simulink model "DisplayModel"  (R2013b)
settings: Solver=FixedStepDiscrete  StartTime=0.0  StopTime=500  FixedStep=1  RelTol=1e-3
PostLoadFcn:
  | clear all;
  | close all;
  | delete(get(0,'Children'));
  | load busdata.mat;
  | load Input_data.mat;
StartFcn:
  | delete(get(0,'Children'));
  | sfcockpitDisplay;
undefined symbols (not defined in the file): AirplaneDirection, AirSpeed, Altitude, APUData, Bearing, CabinPressure, delete, Distance, ECAMInput, EFIS_Pressure, EPR, ExhaustTemp, FlapPosition, FlightAttitude, FuelPressure, FuelQuantity, GroundSpeed, h_ECAM, h_EFIS, h_FCU, h_ND, h_ND_AD, h_PFD_Pages, h_WEng, HydraulicPressure, LandingGear, NDPageInput, OilPressure, RateOfTurn, RPM, SelectedHeading, Temperature, VerticalSpeed
libraries: CockpitDisplayLib x35, aerolibanimutils x1, simulink x1
(part 1 of 2)
settings Model: CovPath=Control_and_Display_Logic/WarningManagement  CovHTMLOptions=-sRT=1 -aTS=1 -bRG=1 -bTC=1 -hTR=0 -nFC=0 -scm=1 -bcm=1 -xEv=0  Creator=siddhars  LastModifiedBy=siddhars
settings DataIOCC: SaveOutput=off  SaveTime=off
settings OptimizationCC: BlockReduction=off  ExpressionDepthLimit=2147483647  OptimizeModelRefInitCode=on  LifeSpan=1
settings DebuggingCC: ArrayBoundsChecking=error  MultiTaskDSMMsg=warning  MultiTaskCondExecSysMsg=none  BusObjectLabelMismatch=error  RootOutportRequireBusObject=error  StateNameClashWarn=warning  NonBusSignalsTreatedAsBus=error
settings RTWCC: SystemTargetFile=ert.tlc  GenCodeOnly=on  TemplateMakefile=ert_default_tmf  Description=Embedded Coder  GenerateReport=on  ProcessScript=ert_make_rtw_hook  IncludeHyperlinkInReport=on  LaunchReport=on  IncludeERTFirstTime=on  GenerateTraceInfo=on  GenerateTraceReport=on  GenerateTraceReportSl=on  GenerateTraceReportSf=on  GenerateTraceReportEml=on  GenerateWebview=on
settings CodeAppCC: IgnoreCustomStorageClasses=off  CustomSymbolStrType=$N$R$M  InternalIdentifier=Classic  ReqsInCode=on
settings ERTTargetCC: CodeReplacementLibrary=ANSI_C  GenerateSampleERTMain=on  SupportComplex=off  ERTCustomFileTemplate=example_file_process.tlc  EnableDataOwnership=on  MemSecPackage=Simulink
settings ConfigComp: Description=Design Verifier Custom Configuration Component  DVMode=DesignErrorDetection  DVMaxProcessTime=2000  DVModelCoverageObjectives=MCDC  DVMaxTestCaseSteps=1000  DVTestSuiteOptimization=CombinedObjectives (Nonlinear Extended)  DVCovFilter=on  DVDetectIntegerOverflow=off  DVDetectDivisionByZero=off  DVDetectDeadLogic=on  DVSaveReport=on  DVDisplayResultsOnModel=on

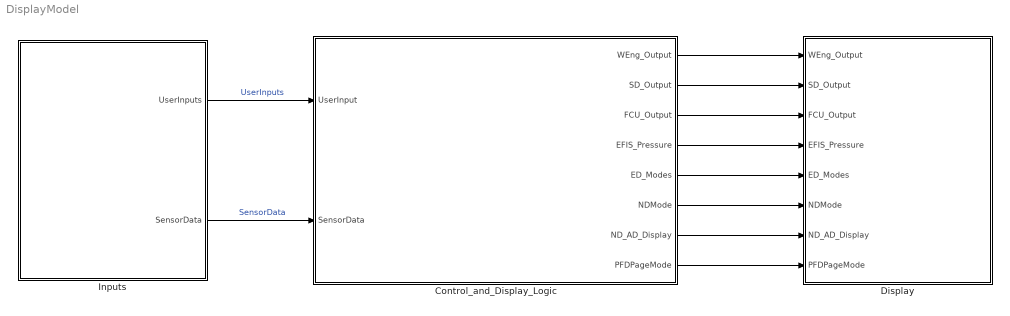
== system DisplayModel ==
  Control_and_Display_Logic : Subsystem  TreatAsAtomicUnit=on
  Display : Subsystem
  Inputs : Subsystem
  wires:
  Inputs/1(UserInputs) -> Control_and_Display_Logic/1(UserInput)  "UserInputs"
  Inputs/2(SensorData) -> Control_and_Display_Logic/2(SensorData)  "SensorData"
  Control_and_Display_Logic/2(SD_Output) -> Display/2(SD_Output)
  Control_and_Display_Logic/7(ND_AD_Display) -> Display/7(ND_AD_Display)
  Control_and_Display_Logic/3(FCU_Output) -> Display/3(FCU_Output)
  Control_and_Display_Logic/1(WEng_Output) -> Display/1(WEng_Output)
  Control_and_Display_Logic/6(NDMode) -> Display/6(NDMode)
  Control_and_Display_Logic/8(PFDPageMode) -> Display/8(PFDPageMode)
  Control_and_Display_Logic/5(ED_Modes) -> Display/5(ED_Modes)
  Control_and_Display_Logic/4(EFIS_Pressure) -> Display/4(EFIS_Pressure)

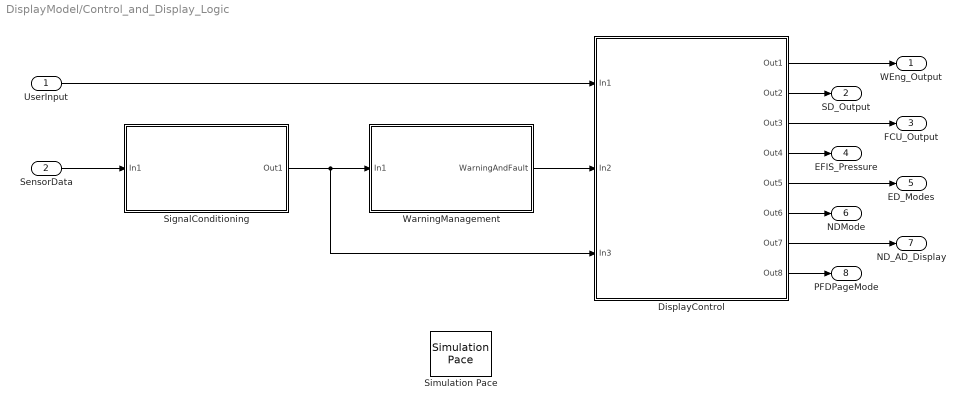
== system DisplayModel/Control_and_Display_Logic ==
  UserInput : Inport
  SensorData : Inport  Port=2
  DisplayControl : Subsystem
  SignalConditioning : Subsystem
  Simulation Pace : aerolibanimutils/Simulation Pace  SimulationPace=4  SleepMode=MATLAB Thread  OutputPaceError=off  SampleTime=1
      settings: AttributesFormatString=%<SimulationPace> sec/sec
  WarningManagement : Subsystem  TreatAsAtomicUnit=on
  WEng_Output : Outport
  SD_Output : Outport  Port=2
  FCU_Output : Outport  Port=3
  EFIS_Pressure : Outport  Port=4
  ED_Modes : Outport  Port=5
  NDMode : Outport  Port=6
  ND_AD_Display : Outport  Port=7
  PFDPageMode : Outport  Port=8
  wires:
  UserInput/1 -> DisplayControl/1(In1)
  SensorData/1 -> SignalConditioning/1(In1)
  SignalConditioning/1(Out1) -> WarningManagement/1(In1), DisplayControl/3(In3)
  DisplayControl/1(Out1) -> WEng_Output/1
  DisplayControl/2(Out2) -> SD_Output/1
  DisplayControl/3(Out3) -> FCU_Output/1
  DisplayControl/4(Out4) -> EFIS_Pressure/1
  DisplayControl/5(Out5) -> ED_Modes/1
  DisplayControl/6(Out6) -> NDMode/1
  DisplayControl/7(Out7) -> ND_AD_Display/1
  DisplayControl/8(Out8) -> PFDPageMode/1
  WarningManagement/1(WarningAndFault) -> DisplayControl/2(In2)

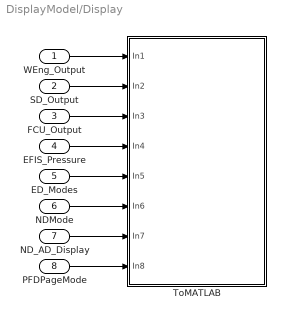
== system DisplayModel/Display ==
  WEng_Output : Inport
  SD_Output : Inport  Port=2
  FCU_Output : Inport  Port=3
  EFIS_Pressure : Inport  Port=4
  ED_Modes : Inport  Port=5
  NDMode : Inport  Port=6
  ND_AD_Display : Inport  Port=7
  PFDPageMode : Inport  Port=8
  ToMATLAB : Subsystem
  wires:
  PFDPageMode/1 -> ToMATLAB/8(In8)
  ND_AD_Display/1 -> ToMATLAB/7(In7)
  NDMode/1 -> ToMATLAB/6(In6)
  ED_Modes/1 -> ToMATLAB/5(In5)
  EFIS_Pressure/1 -> ToMATLAB/4(In4)
  FCU_Output/1 -> ToMATLAB/3(In3)
  SD_Output/1 -> ToMATLAB/2(In2)
  WEng_Output/1 -> ToMATLAB/1(In1)

== system DisplayModel/Inputs ==
  Sensors : Subsystem
  UserSelection : Subsystem
  UserInputs : Outport
  SensorData : Outport  Port=2
  wires:
  UserSelection/1(Out1) -> UserInputs/1
  UserSelection/2(Out2) -> Sensors/1(PowerSwitch)
  Sensors/1(SensorData) -> SensorData/1

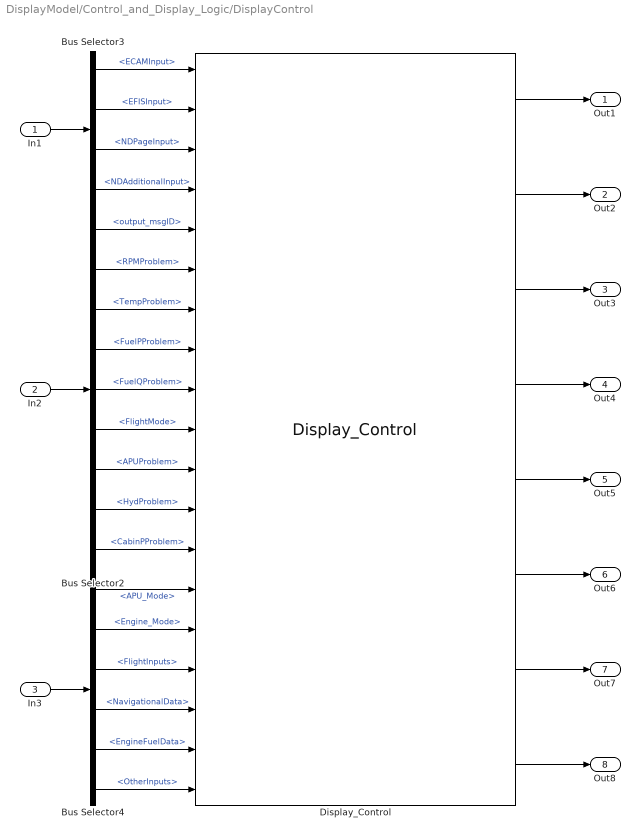
== system DisplayModel/Control_and_Display_Logic/DisplayControl ==
  In1 : Inport
  In2 : Inport  Port=2
  In3 : Inport  Port=3
  Bus Selector2 : BusSelector  OutputSignals=output_msgID,RPMProblem,TempProblem,FuelPProblem,FuelQProblem,FlightMode,APUProblem,HydProblem,CabinPProblem
  Bus Selector3 : BusSelector  OutputSignals=ECAMInput,EFISInput,NDPageInput,NDAdditionalInput
  Bus Selector4 : BusSelector  OutputSignals=EnergySystemModes.APU_Mode,EnergySystemModes.Engine_Mode,FlightInputs,NavigationalData,EngineFuelData,OtherInputs
  Display_Control : CockpitDisplayLib/Display_Control  SystemSampleTime=-1
  Out1 : Outport
  Out2 : Outport  Port=2
  Out3 : Outport  Port=3
  Out4 : Outport  Port=4
  Out5 : Outport  Port=5
  Out6 : Outport  Port=6
  Out7 : Outport  Port=7
  Out8 : Outport  Port=8
  wires:
  In2/1 -> Bus Selector2/1
  In3/1 -> Bus Selector4/1
  In1/1 -> Bus Selector3/1
  Bus Selector2/4 -> Display_Control/8  "<FuelPProblem>"
  Bus Selector2/3 -> Display_Control/7  "<TempProblem>"
  Display_Control/1 -> Out1/1
  Bus Selector2/8 -> Display_Control/12  "<HydProblem>"
  Bus Selector2/5 -> Display_Control/9  "<FuelQProblem>"
  Display_Control/8 -> Out8/1
  Display_Control/6 -> Out6/1
  Bus Selector2/6 -> Display_Control/10  "<FlightMode>"
  Bus Selector3/1 -> Display_Control/1  "<ECAMInput>"
  Display_Control/4 -> Out4/1
  Display_Control/3 -> Out3/1
  Bus Selector2/9 -> Display_Control/13  "<CabinPProblem>"
  Bus Selector3/2 -> Display_Control/2  "<EFISInput>"
  Display_Control/2 -> Out2/1
  Bus Selector2/2 -> Display_Control/6  "<RPMProblem>"
  Bus Selector3/3 -> Display_Control/3  "<NDPageInput>"
  Bus Selector3/4 -> Display_Control/4  "<NDAdditionalInput>"
  Bus Selector2/7 -> Display_Control/11  "<APUProblem>"
  Bus Selector2/1 -> Display_Control/5  "<output_msgID>"
  Display_Control/5 -> Out5/1
  Display_Control/7 -> Out7/1
  Bus Selector4/6 -> Display_Control/19  "<OtherInputs>"
  Bus Selector4/5 -> Display_Control/18  "<EngineFuelData>"
  Bus Selector4/4 -> Display_Control/17  "<NavigationalData>"
  Bus Selector4/3 -> Display_Control/16  "<FlightInputs>"
  Bus Selector4/2 -> Display_Control/15  "<Engine_Mode>"
  Bus Selector4/1 -> Display_Control/14  "<APU_Mode>"

== system DisplayModel/Control_and_Display_Logic/SignalConditioning ==
  In1 : Inport
  Bus Creator1 : BusCreator  Inputs=5
  Bus Selector6 : BusSelector  OutputSignals=EnergySystemModes,FlightInputs,NavigationalData,EngineFuelData,OtherInputs
  SignalSelection : Subsystem
  Out1 : Outport
  wires:
  Bus Selector6/2 -> Bus Creator1/2  "<FlightInputs>"
  Bus Creator1/1 -> Out1/1
  Bus Selector6/5 -> SignalSelection/2(In2)  "<OtherInputs>"
  Bus Selector6/4 -> SignalSelection/1(In1)  "<EngineFuelData>"
  Bus Selector6/3 -> Bus Creator1/3  "<NavigationalData>"
  SignalSelection/1(Out1) -> Bus Creator1/4  "EngineFuelData"
  In1/1 -> Bus Selector6/1
  SignalSelection/2(Out2) -> Bus Creator1/5  "OtherInputs"
  Bus Selector6/1 -> Bus Creator1/1  "<EnergySystemModes>"

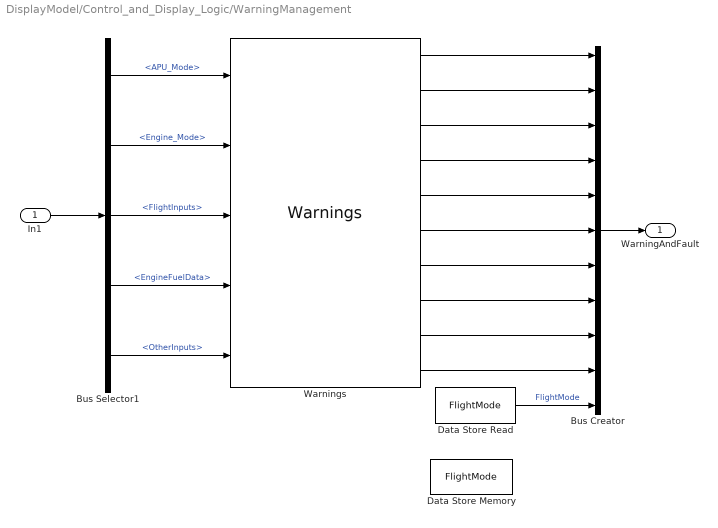
== system DisplayModel/Control_and_Display_Logic/WarningManagement ==
  In1 : Inport
  Bus Creator : BusCreator  Inputs=11
  Bus Selector1 : BusSelector  OutputSignals=EnergySystemModes.APU_Mode,EnergySystemModes.Engine_Mode,FlightInputs,EngineFuelData,OtherInputs
  Data Store Memory : DataStoreMemory  DataStoreName=FlightMode  ReadBeforeWriteMsg=warning  WriteAfterWriteMsg=warning  WriteAfterReadMsg=warning  OutDataTypeStr=double  Dimensions=1
  Data Store Read : DataStoreRead  Priority=1  DataStoreName=FlightMode  SampleTime=1
  Warnings : CockpitDisplayLib/Warnings  Priority=0  SystemSampleTime=-1
  WarningAndFault : Outport
  wires:
  In1/1 -> Bus Selector1/1
  Bus Creator/1 -> WarningAndFault/1
  Warnings/3 -> Bus Creator/3
  Warnings/6 -> Bus Creator/6
  Warnings/5 -> Bus Creator/5
  Warnings/4 -> Bus Creator/4
  Warnings/9 -> Bus Creator/9
  Warnings/7 -> Bus Creator/7
  Warnings/1 -> Bus Creator/1
  Warnings/10 -> Bus Creator/10
  Warnings/8 -> Bus Creator/8
  Warnings/2 -> Bus Creator/2
  Data Store Read/1 -> Bus Creator/11  "FlightMode"
  Bus Selector1/5 -> Warnings/5  "<OtherInputs>"
  Bus Selector1/4 -> Warnings/4  "<EngineFuelData>"
  Bus Selector1/3 -> Warnings/3  "<FlightInputs>"
  Bus Selector1/1 -> Warnings/1  "<APU_Mode>"
  Bus Selector1/2 -> Warnings/2  "<Engine_Mode>"

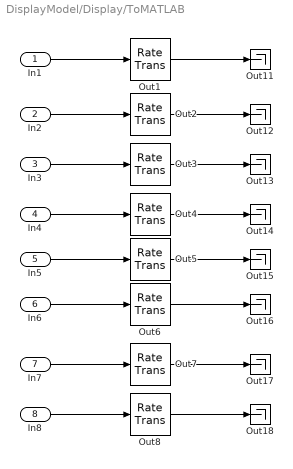
== system DisplayModel/Display/ToMATLAB ==
  In1 : Inport
  In2 : Inport  Port=2
  In3 : Inport  Port=3
  In4 : Inport  Port=4
  In5 : Inport  Port=5
  In6 : Inport  Port=6
  In7 : Inport  Port=7
  In8 : Inport  Port=8
  Out1 : RateTransition  StartFcn=|  StopFcn=delete(h_WEng)
      | blk='DisplayModel/Display/ToMATLAB/Out1';                                  
      | h_WEng=add_exec_event_listener(blk,'PostOutputs',@sfCockpitDisplay_helper);
  Out{11..18} (8 alike) : Terminator
  Out2 : RateTransition  StartFcn=|  StopFcn=delete(h_ECAM)
      | blk='DisplayModel/Display/ToMATLAB/Out2';                                  
      | h_ECAM=add_exec_event_listener(blk,'PostOutputs',@sfCockpitDisplay_helper);
  Out3 : RateTransition  StartFcn=|  StopFcn=delete(h_FCU)
      | blk='DisplayModel/Display/ToMATLAB/Out3';                                 
      | h_FCU=add_exec_event_listener(blk,'PostOutputs',@sfCockpitDisplay_helper);
  Out4 : RateTransition  StartFcn=|  StopFcn=delete(h_EFIS)
      | blk='DisplayModel/Display/ToMATLAB/Out4';                                  
      | h_EFIS=add_exec_event_listener(blk,'PostOutputs',@sfCockpitDisplay_helper);
  Out5 : RateTransition  StartFcn=|  StopFcn=|
      StartFcn=|
      | blk='DisplayModel/Display/ToMATLAB/Out5';                                  
      | h_ED_L=add_exec_event_listener(blk,'PostOutputs',@sfCockpitDisplay_helper);
      |                                                                            
      | h_ED_R=add_exec_event_listener(blk,'PostOutputs',@sfCockpitDisplay_helper);
      StopFcn=|
      | delete(h_ED_L)
      | delete(h_ED_R)
  Out6 : RateTransition  StartFcn=|  StopFcn=delete(h_ND)
      | blk='DisplayModel/Display/ToMATLAB/Out6';                                
      | h_ND=add_exec_event_listener(blk,'PostOutputs',@sfCockpitDisplay_helper);
  Out7 : RateTransition  StartFcn=|  StopFcn=delete(h_ND_AD)
      | blk='DisplayModel/Display/ToMATLAB/Out7';                                   
      | h_ND_AD=add_exec_event_listener(blk,'PostOutputs',@sfCockpitDisplay_helper);
  Out8 : RateTransition  StartFcn=|  StopFcn=delete(h_PFD_Pages)
      | blk='DisplayModel/Display/ToMATLAB/Out8';                                       
      | h_PFD_Pages=add_exec_event_listener(blk,'PostOutputs',@sfCockpitDisplay_helper);
  wires:
  Out1/1 -> Out11/1
  Out7/1 -> Out17/1
  Out5/1 -> Out15/1
  Out8/1 -> Out18/1
  Out6/1 -> Out16/1
  Out3/1 -> Out13/1
  Out2/1 -> Out12/1
  Out4/1 -> Out14/1
  In2/1 -> Out2/1
  In1/1 -> Out1/1
  In8/1 -> Out8/1
  In7/1 -> Out7/1
  In6/1 -> Out6/1
  In5/1 -> Out5/1
  In4/1 -> Out4/1
  In3/1 -> Out3/1

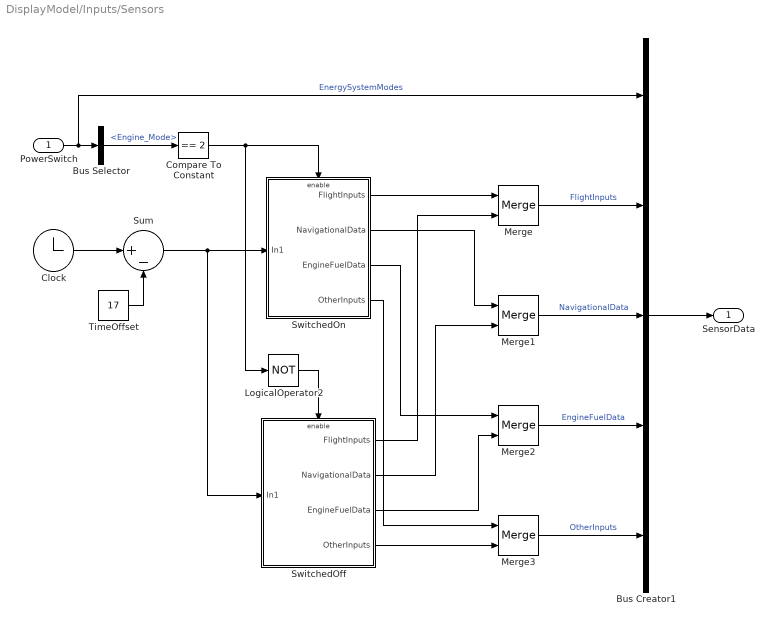
== system DisplayModel/Inputs/Sensors ==
  PowerSwitch : Inport
  Bus Creator1 : BusCreator  Inputs=5
  Bus Selector : BusSelector  OutputSignals=Engine_Mode
  Clock : Clock
  Compare To Constant : simulink/Logic and Bit Operations/Compare To Constant  relop===  const=2  OutDataTypeStr=boolean
  LogicalOperator2 : Logic  Operator=NOT  AllPortsSameDT=off  OutDataTypeStr=boolean
  Merge{,1..3} (4 alike) : Merge
  Sum : Sum  Inputs=|+-
  SwitchedOff : Subsystem
  SwitchedOn : Subsystem
  TimeOffset : Constant  Value=17
  SensorData : Outport
  wires:
  Clock/1 -> Sum/1
  Merge/1 -> Bus Creator1/2  "FlightInputs"
  SwitchedOff/1(FlightInputs) -> Merge/2
  SwitchedOn/4("OtherInputs ") -> Merge3/1
  SwitchedOff/3(EngineFuelData) -> Merge2/2
  SwitchedOff/2("NavigationalData ") -> Merge1/2
  SwitchedOn/1(FlightInputs) -> Merge/1
  SwitchedOn/2("NavigationalData ") -> Merge1/1
  Merge1/1 -> Bus Creator1/3  "NavigationalData"
  SwitchedOff/4("OtherInputs ") -> Merge3/2
  SwitchedOn/3(EngineFuelData) -> Merge2/1
  TimeOffset/1 -> Sum/2
  Sum/1 -> SwitchedOn/1(In1), SwitchedOff/1(In1)
  LogicalOperator2/1 -> SwitchedOff/Enable
  Bus Creator1/1 -> SensorData/1
  Merge2/1 -> Bus Creator1/4  "EngineFuelData"
  Merge3/1 -> Bus Creator1/5  "OtherInputs"
  PowerSwitch/1 -> Bus Selector/1, Bus Creator1/1  "EnergySystemModes"
  Bus Selector/1 -> Compare To Constant/1  "<Engine_Mode>"
  Compare To Constant/1 -> LogicalOperator2/1, SwitchedOn/Enable

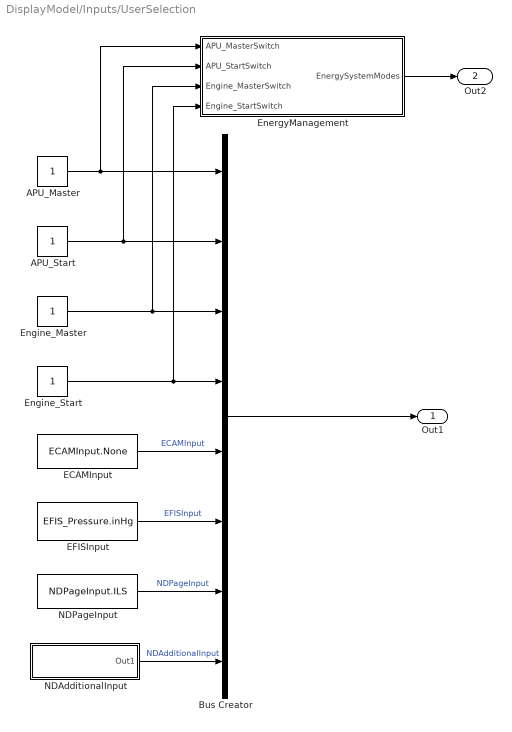
== system DisplayModel/Inputs/UserSelection ==
  APU_Master : Constant  OutDataTypeStr=boolean
  APU_Start : Constant  OutDataTypeStr=boolean
  Bus Creator : BusCreator  Inputs=8
  ECAMInput : Constant  Value=ECAMInput.None  OutDataTypeStr=Enum: ECAMInput
  EFISInput : Constant  Value=EFIS_Pressure.inHg  OutDataTypeStr=Enum: EFIS_Pressure
  EnergyManagement : Subsystem
  Engine_Master : Constant  OutDataTypeStr=boolean
  Engine_Start : Constant  OutDataTypeStr=boolean
  NDAdditionalInput : Subsystem
  NDPageInput : Constant  Value=NDPageInput.ILS  OutDataTypeStr=Enum: NDPageInput
  Out1 : Outport
  Out2 : Outport  Port=2
  wires:
  APU_Start/1 -> Bus Creator/2, EnergyManagement/2(APU_StartSwitch)
  Engine_Start/1 -> Bus Creator/4, EnergyManagement/4(Engine_StartSwitch)
  Engine_Master/1 -> Bus Creator/3, EnergyManagement/3(Engine_MasterSwitch)
  EFISInput/1 -> Bus Creator/6  "EFISInput"
  ECAMInput/1 -> Bus Creator/5  "ECAMInput"
  APU_Master/1 -> Bus Creator/1, EnergyManagement/1(APU_MasterSwitch)
  NDPageInput/1 -> Bus Creator/7  "NDPageInput"
  NDAdditionalInput/1(Out1) -> Bus Creator/8  "NDAdditionalInput"
  Bus Creator/1 -> Out1/1
  EnergyManagement/1(EnergySystemModes) -> Out2/1

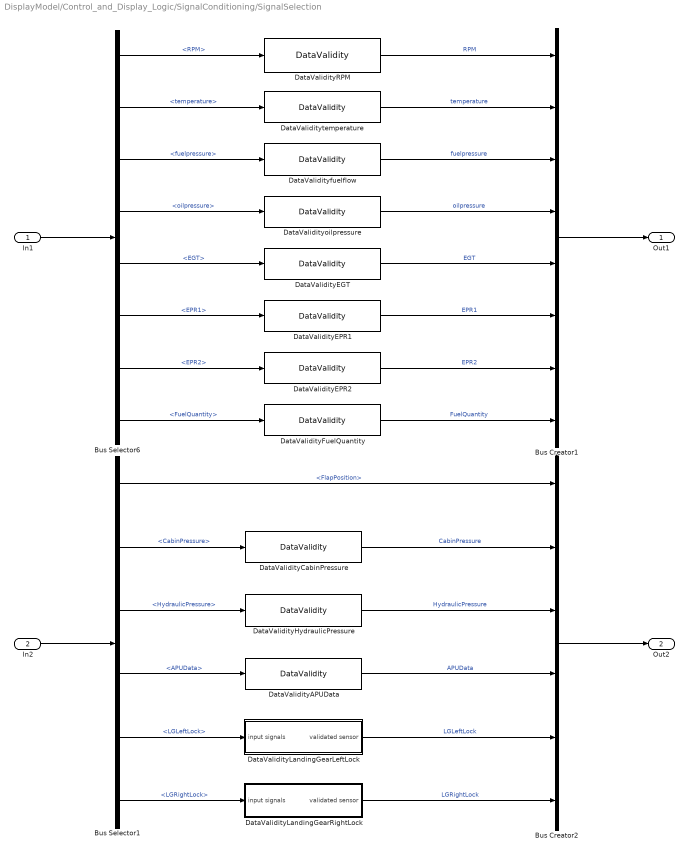
== system DisplayModel/Control_and_Display_Logic/SignalConditioning/SignalSelection ==
  In1 : Inport
  In2 : Inport  Port=2
  Bus Creator1 : BusCreator  Inputs=8  OutDataTypeStr=Bus: EngineFuel_Bus
  Bus Creator2 : BusCreator  Inputs=6  OutDataTypeStr=Bus: MiscData
  Bus Selector1 : BusSelector  OutputSignals=FlapPosition,CabinPressure,HydraulicPressure,APUData,LGLeftLock,LGRightLock
  Bus Selector6 : BusSelector  OutputSignals=RPM,temperature,fuelpressure,oilpressure,EGT,EPR1,EPR2,FuelQuantity
  DataValidityAPUData : CockpitDisplayLib/DataValidity
  DataValidityCabinPressure : CockpitDisplayLib/DataValidity
  DataValidityEGT : CockpitDisplayLib/DataValidity
  DataValidityEPR1 : CockpitDisplayLib/DataValidity
  DataValidityEPR2 : CockpitDisplayLib/DataValidity
  DataValidityFuelQuantity : CockpitDisplayLib/DataValidity
  DataValidityHydraulicPressure : CockpitDisplayLib/DataValidity
  DataValidityLandingGearLeftLock : Subsystem
  DataValidityLandingGearRightLock : Subsystem
  DataValidityRPM : CockpitDisplayLib/DataValidity
  DataValidityfuelflow : CockpitDisplayLib/DataValidity
  DataValidityoilpressure : CockpitDisplayLib/DataValidity
  DataValiditytemperature : CockpitDisplayLib/DataValidity
  Out1 : Outport
  Out2 : Outport  Port=2  OutDataTypeStr=Bus: MiscData
  wires:
  Bus Selector6/1 -> DataValidityRPM/1  "<RPM>"
  Bus Creator1/1 -> Out1/1
  DataValidityRPM/1 -> Bus Creator1/1  "RPM"
  Bus Selector6/6 -> DataValidityEPR1/1  "<EPR1>"
  In1/1 -> Bus Selector6/1
  Bus Selector6/4 -> DataValidityoilpressure/1  "<oilpressure>"
  Bus Selector6/5 -> DataValidityEGT/1  "<EGT>"
  Bus Selector6/3 -> DataValidityfuelflow/1  "<fuelpressure>"
  Bus Selector6/7 -> DataValidityEPR2/1  "<EPR2>"
  DataValidityoilpressure/1 -> Bus Creator1/4  "oilpressure"
  DataValidityfuelflow/1 -> Bus Creator1/3  "fuelpressure"
  DataValiditytemperature/1 -> Bus Creator1/2  "temperature"
  Bus Selector6/2 -> DataValiditytemperature/1  "<temperature>"
  In2/1 -> Bus Selector1/1
  Bus Creator2/1 -> Out2/1
  Bus Selector1/1 -> Bus Creator2/1  "<FlapPosition>"
  Bus Selector1/2 -> DataValidityCabinPressure/1  "<CabinPressure>"
  Bus Selector1/3 -> DataValidityHydraulicPressure/1  "<HydraulicPressure>"
  Bus Selector1/4 -> DataValidityAPUData/1  "<APUData>"
  Bus Selector1/5 -> DataValidityLandingGearLeftLock/1(input signals)  "<LGLeftLock>"
  DataValidityCabinPressure/1 -> Bus Creator2/2  "CabinPressure"
  DataValidityHydraulicPressure/1 -> Bus Creator2/3  "HydraulicPressure"
  DataValidityAPUData/1 -> Bus Creator2/4  "APUData"
  DataValidityLandingGearLeftLock/1(validated sensor) -> Bus Creator2/5  "LGLeftLock"
  DataValidityEGT/1 -> Bus Creator1/5  "EGT"
  DataValidityEPR1/1 -> Bus Creator1/6  "EPR1"
  DataValidityEPR2/1 -> Bus Creator1/7  "EPR2"
  Bus Selector6/8 -> DataValidityFuelQuantity/1  "<FuelQuantity>"
  DataValidityFuelQuantity/1 -> Bus Creator1/8  "FuelQuantity"
  DataValidityLandingGearRightLock/1(validated sensor) -> Bus Creator2/6  "LGRightLock"
  Bus Selector1/6 -> DataValidityLandingGearRightLock/1(input signals)  "<LGRightLock>"

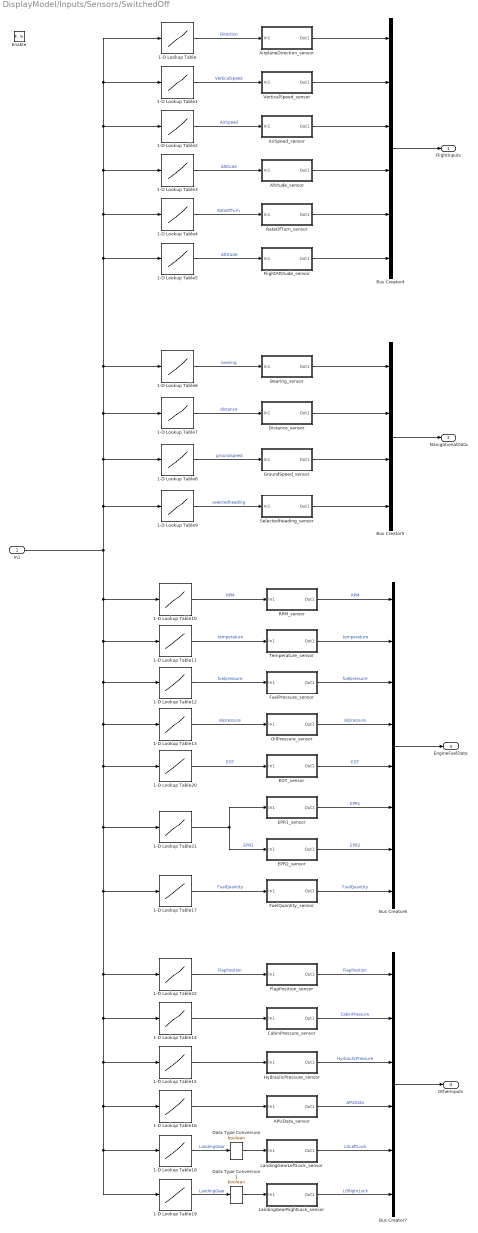
== system DisplayModel/Inputs/Sensors/SwitchedOff ==
  In1 : Inport
  Enable : EnablePort
  1-D Lookup Table{,1..17,20..22} (21 alike) : Lookup_n-D  NumberOfTableDimensions=1  BreakpointsForDimension1=0:10:500  Table=zeros(51,1)  RndMeth=Simplest  InputSameDT=on
  1-D Lookup Table18 : Lookup_n-D  NumberOfTableDimensions=1  BreakpointsForDimension1=0:10:500  Table=ones(51,1)  RndMeth=Simplest  InputSameDT=on
  1-D Lookup Table19 : Lookup_n-D  NumberOfTableDimensions=1  BreakpointsForDimension1=0:10:500  Table=ones(51,1)  RndMeth=Simplest  InputSameDT=on
  APUData_sensor : Subsystem
  AirSpeed_sensor : Subsystem
  AirplaneDirection_sensor : Subsystem
  Altitude_sensor : Subsystem
  Bearing_sensor : Subsystem
  Bus Creator4 : BusCreator  Inputs=6  OutDataTypeStr=Bus: FlightInputs
  Bus Creator5 : BusCreator  OutDataTypeStr=Bus: NavData
  Bus Creator6 : BusCreator  Inputs='RPM','temperature','fuelpressure','oilpressure','EGT','EPR1','EPR2','FuelQuantity'  OutDataTypeStr=Bus: IN_EngineFuel_Bus
  Bus Creator7 : BusCreator  Inputs=6  OutDataTypeStr=Bus: IN_MiscData
  CabinPressure_sensor : Subsystem
  Data Type Conversion : DataTypeConversion  OutDataTypeStr=boolean
  Data Type Conversion1 : DataTypeConversion  OutDataTypeStr=boolean
  Distance_sensor : Subsystem
  EGT_sensor : Subsystem
  EPR1_sensor : Subsystem
  EPR2_sensor : Subsystem
  FlapPosition_sensor : Subsystem
  FlightAttitude_sensor : Subsystem
  FuelPressure_sensor : Subsystem
  FuelQuantity_sensor : Subsystem
  GroundSpeed_sensor : Subsystem
  HydraulicPressure_sensor : Subsystem
  LandingGearLeftLock_sensor : Subsystem
  LandingGearRightLock_sensor : Subsystem
  OilPressure_sensor : Subsystem
  RPM_sensor : Subsystem
  RateOfTurn_sensor : Subsystem
  SelectedHeading_sensor : Subsystem
  Temperature_sensor : Subsystem
  VerticalSpeed_sensor : Subsystem
  FlightInputs : Outport
  "NavigationalData " : Outport  Port=2
  EngineFuelData : Outport  Port=3
  "OtherInputs " : Outport  Port=4
  wires:
  Bus Creator7/1 -> "OtherInputs "/1
  1-D Lookup Table22/1 -> FlapPosition_sensor/1(In1)  "FlapPosition"
  Bus Creator6/1 -> EngineFuelData/1
  1-D Lookup Table11/1 -> Temperature_sensor/1(In1)  "temperature"
  Bus Creator5/1 -> "NavigationalData "/1
  1-D Lookup Table9/1 -> SelectedHeading_sensor/1(In1)  "selectedheading"
  1-D Lookup Table8/1 -> GroundSpeed_sensor/1(In1)  "groundspeed"
  1-D Lookup Table6/1 -> Bearing_sensor/1(In1)  "bearing"
  1-D Lookup Table7/1 -> Distance_sensor/1(In1)  "distance"
  Bus Creator4/1 -> FlightInputs/1
  1-D Lookup Table5/1 -> FlightAttitude_sensor/1(In1)  "Attitude"
  1-D Lookup Table4/1 -> RateOfTurn_sensor/1(In1)  "RateOfTurn"
  1-D Lookup Table/1 -> AirplaneDirection_sensor/1(In1)  "Direction"
  1-D Lookup Table3/1 -> Altitude_sensor/1(In1)  "Altitude"
  1-D Lookup Table1/1 -> VerticalSpeed_sensor/1(In1)  "VerticalSpeed"
  1-D Lookup Table2/1 -> AirSpeed_sensor/1(In1)  "AirSpeed"
  1-D Lookup Table20/1 -> EGT_sensor/1(In1)  "EGT"
  1-D Lookup Table14/1 -> CabinPressure_sensor/1(In1)
  CabinPressure_sensor/1(Out1) -> Bus Creator7/2  "CabinPressure"
  1-D Lookup Table18/1 -> Data Type Conversion/1  "LandingGear"
  LandingGearLeftLock_sensor/1(Out1) -> Bus Creator7/5  "LGLeftLock"
  1-D Lookup Table16/1 -> APUData_sensor/1(In1)
  APUData_sensor/1(Out1) -> Bus Creator7/4  "APUData"
  1-D Lookup Table15/1 -> HydraulicPressure_sensor/1(In1)
  HydraulicPressure_sensor/1(Out1) -> Bus Creator7/3  "HydraulicPressure"
  EPR1_sensor/1(Out1) -> Bus Creator6/6  "EPR1"
  1-D Lookup Table13/1 -> OilPressure_sensor/1(In1)  "oilpressure"
  OilPressure_sensor/1(Out1) -> Bus Creator6/4  "oilpressure"
  1-D Lookup Table12/1 -> FuelPressure_sensor/1(In1)  "fuelpressure"
  FuelPressure_sensor/1(Out1) -> Bus Creator6/3  "fuelpressure"
  1-D Lookup Table10/1 -> RPM_sensor/1(In1)  "RPM"
  RPM_sensor/1(Out1) -> Bus Creator6/1  "RPM"
  Temperature_sensor/1(Out1) -> Bus Creator6/2  "temperature"
  SelectedHeading_sensor/1(Out1) -> Bus Creator5/4
  GroundSpeed_sensor/1(Out1) -> Bus Creator5/3
  Distance_sensor/1(Out1) -> Bus Creator5/2
  Bearing_sensor/1(Out1) -> Bus Creator5/1
  FlightAttitude_sensor/1(Out1) -> Bus Creator4/6
  RateOfTurn_sensor/1(Out1) -> Bus Creator4/5
  Altitude_sensor/1(Out1) -> Bus Creator4/4
  AirSpeed_sensor/1(Out1) -> Bus Creator4/3
  VerticalSpeed_sensor/1(Out1) -> Bus Creator4/2
  AirplaneDirection_sensor/1(Out1) -> Bus Creator4/1
  EGT_sensor/1(Out1) -> Bus Creator6/5  "EGT"
  FlapPosition_sensor/1(Out1) -> Bus Creator7/1  "FlapPosition"
  1-D Lookup Table21/1 -> EPR1_sensor/1(In1), EPR2_sensor/1(In1)  "EPR1"
  EPR2_sensor/1(Out1) -> Bus Creator6/7  "EPR2"
  1-D Lookup Table17/1 -> FuelQuantity_sensor/1(In1)  "FuelQuantity"
  FuelQuantity_sensor/1(Out1) -> Bus Creator6/8  "FuelQuantity"
  Data Type Conversion/1 -> LandingGearLeftLock_sensor/1(In1)
  1-D Lookup Table19/1 -> Data Type Conversion1/1  "LandingGear"
  LandingGearRightLock_sensor/1(Out1) -> Bus Creator7/6  "LGRightLock"
  In1/1 -> 1-D Lookup Table17/1, 1-D Lookup Table18/1, 1-D Lookup Table19/1, 1-D Lookup Table16/1, 1-D Lookup Table15/1, 1-D Lookup Table14/1, 1-D Lookup Table22/1, 1-D Lookup Table21/1, 1-D Lookup Table20/1, 1-D Lookup Table13/1, 1-D Lookup Table12/1, 1-D Lookup Table11/1, 1-D Lookup Table10/1, 1-D Lookup Table5/1, 1-D Lookup Table3/1, 1-D Lookup Table2/1, 1-D Lookup Table1/1, 1-D Lookup Table/1, 1-D Lookup Table4/1, 1-D Lookup Table6/1, 1-D Lookup Table7/1, 1-D Lookup Table8/1, 1-D Lookup Table9/1
  Data Type Conversion1/1 -> LandingGearRightLock_sensor/1(In1)

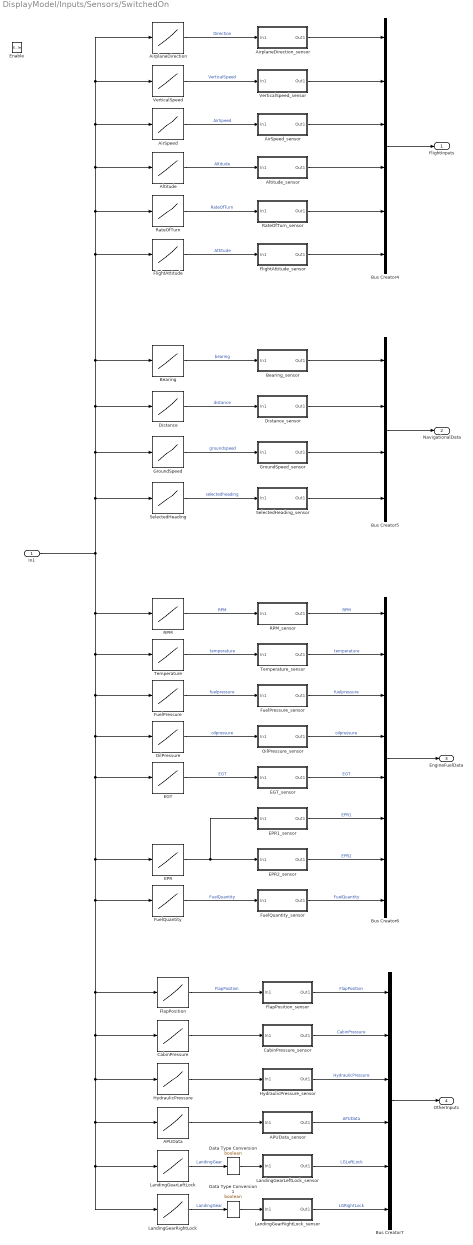
== system DisplayModel/Inputs/Sensors/SwitchedOn ==
  In1 : Inport
  Enable : EnablePort
  APUData : Lookup_n-D  NumberOfTableDimensions=1  BreakpointsForDimension1=0:10:500  Table=APUData  RndMeth=Simplest  InputSameDT=on
  APUData_sensor : Subsystem
  AirSpeed : Lookup_n-D  NumberOfTableDimensions=1  BreakpointsForDimension1=0:10:500  Table=AirSpeed  RndMeth=Simplest  InputSameDT=on
  AirSpeed_sensor : Subsystem
  AirplaneDirection : Lookup_n-D  NumberOfTableDimensions=1  BreakpointsForDimension1=0:10:500  Table=AirplaneDirection  RndMeth=Simplest  InputSameDT=on
  AirplaneDirection_sensor : Subsystem
  Altitude : Lookup_n-D  NumberOfTableDimensions=1  BreakpointsForDimension1=0:10:500  Table=Altitude  RndMeth=Simplest  InputSameDT=on
  Altitude_sensor : Subsystem
  Bearing : Lookup_n-D  NumberOfTableDimensions=1  BreakpointsForDimension1=0:10:500  Table=Bearing  RndMeth=Simplest  InputSameDT=on
  Bearing_sensor : Subsystem
  Bus Creator4 : BusCreator  Inputs=6  OutDataTypeStr=Bus: FlightInputs
  Bus Creator5 : BusCreator  OutDataTypeStr=Bus: NavData
  Bus Creator6 : BusCreator  Inputs=8  OutDataTypeStr=Bus: IN_EngineFuel_Bus
  Bus Creator7 : BusCreator  Inputs=6  OutDataTypeStr=Bus: IN_MiscData
  CabinPressure : Lookup_n-D  NumberOfTableDimensions=1  BreakpointsForDimension1=0:10:500  Table=CabinPressure  RndMeth=Simplest  InputSameDT=on
  CabinPressure_sensor : Subsystem
  Data Type Conversion : DataTypeConversion  OutDataTypeStr=boolean
  Data Type Conversion1 : DataTypeConversion  OutDataTypeStr=boolean
  Distance : Lookup_n-D  NumberOfTableDimensions=1  BreakpointsForDimension1=0:10:500  Table=Distance  RndMeth=Simplest  InputSameDT=on
  Distance_sensor : Subsystem
  EGT : Lookup_n-D  NumberOfTableDimensions=1  BreakpointsForDimension1=0:1:500  Table=ExhaustTemp  RndMeth=Simplest  InputSameDT=on
  EGT_sensor : Subsystem
  EPR : Lookup_n-D  NumberOfTableDimensions=1  BreakpointsForDimension1=0:10:500  Table=EPR  RndMeth=Simplest  InputSameDT=on
  EPR1_sensor : Subsystem
  EPR2_sensor : Subsystem
  "FlapPosition " : Lookup_n-D  NumberOfTableDimensions=1  BreakpointsForDimension1=0:10:500  Table=FlapPosition  RndMeth=Simplest  InputSameDT=on
  FlapPosition_sensor : Subsystem
  FlightAttitude : Lookup_n-D  NumberOfTableDimensions=1  BreakpointsForDimension1=0:10:500  Table=FlightAttitude  RndMeth=Simplest  InputSameDT=on
  FlightAttitude_sensor : Subsystem
  FuelPressure : Lookup_n-D  NumberOfTableDimensions=1  BreakpointsForDimension1=0:10:500  Table=FuelPressure  RndMeth=Simplest  InputSameDT=on
  FuelPressure_sensor : Subsystem
  FuelQuantity : Lookup_n-D  NumberOfTableDimensions=1  BreakpointsForDimension1=0:10:500  Table=FuelQuantity  RndMeth=Simplest  InputSameDT=on
  FuelQuantity_sensor : Subsystem
  GroundSpeed : Lookup_n-D  NumberOfTableDimensions=1  BreakpointsForDimension1=0:10:500  Table=GroundSpeed  RndMeth=Simplest  InputSameDT=on
  GroundSpeed_sensor : Subsystem
  HydraulicPressure : Lookup_n-D  NumberOfTableDimensions=1  BreakpointsForDimension1=0:10:500  Table=HydraulicPressure  RndMeth=Simplest  InputSameDT=on
  HydraulicPressure_sensor : Subsystem
  LandingGearLeftLock : Lookup_n-D  NumberOfTableDimensions=1  BreakpointsForDimension1=0:10:500  Table=LandingGear  RndMeth=Simplest  InputSameDT=on
  LandingGearLeftLock_sensor : Subsystem
  LandingGearRightLock : Lookup_n-D  NumberOfTableDimensions=1  BreakpointsForDimension1=0:10:500  Table=LandingGear  RndMeth=Simplest  InputSameDT=on
  LandingGearRightLock_sensor : Subsystem
  OilPressure : Lookup_n-D  NumberOfTableDimensions=1  BreakpointsForDimension1=0:10:500  Table=OilPressure  RndMeth=Simplest  InputSameDT=on
  OilPressure_sensor : Subsystem
  RPM : Lookup_n-D  NumberOfTableDimensions=1  BreakpointsForDimension1=0:10:500  Table=RPM  RndMeth=Simplest  InputSameDT=on
  RPM_sensor : Subsystem
  RateOfTurn : Lookup_n-D  NumberOfTableDimensions=1  BreakpointsForDimension1=0:10:500  Table=RateOfTurn  RndMeth=Simplest  InputSameDT=on
  RateOfTurn_sensor : Subsystem
  SelectedHeading : Lookup_n-D  NumberOfTableDimensions=1  BreakpointsForDimension1=0:10:500  Table=SelectedHeading  RndMeth=Simplest  InputSameDT=on
  SelectedHeading_sensor : Subsystem
  Temperature : Lookup_n-D  NumberOfTableDimensions=1  BreakpointsForDimension1=0:10:500  Table=Temperature  RndMeth=Simplest  InputSameDT=on
  Temperature_sensor : Subsystem
  VerticalSpeed : Lookup_n-D  NumberOfTableDimensions=1  BreakpointsForDimension1=0:10:500  Table=VerticalSpeed  RndMeth=Simplest  InputSameDT=on
  VerticalSpeed_sensor : Subsystem
  FlightInputs : Outport
  "NavigationalData " : Outport  Port=2
  EngineFuelData : Outport  Port=3
  "OtherInputs " : Outport  Port=4
  wires:
  Bus Creator7/1 -> "OtherInputs "/1
  "FlapPosition "/1 -> FlapPosition_sensor/1(In1)  "FlapPosition"
  Bus Creator6/1 -> EngineFuelData/1
  Temperature/1 -> Temperature_sensor/1(In1)  "temperature"
  Bus Creator5/1 -> "NavigationalData "/1
  SelectedHeading/1 -> SelectedHeading_sensor/1(In1)  "selectedheading"
  GroundSpeed/1 -> GroundSpeed_sensor/1(In1)  "groundspeed"
  Bearing/1 -> Bearing_sensor/1(In1)  "bearing"
  Distance/1 -> Distance_sensor/1(In1)  "distance"
  Bus Creator4/1 -> FlightInputs/1
  FlightAttitude/1 -> FlightAttitude_sensor/1(In1)  "Attitude"
  RateOfTurn/1 -> RateOfTurn_sensor/1(In1)  "RateOfTurn"
  AirplaneDirection/1 -> AirplaneDirection_sensor/1(In1)  "Direction"
  Altitude/1 -> Altitude_sensor/1(In1)  "Altitude"
  VerticalSpeed/1 -> VerticalSpeed_sensor/1(In1)  "VerticalSpeed"
  AirSpeed/1 -> AirSpeed_sensor/1(In1)  "AirSpeed"
  EPR/1 -> EPR1_sensor/1(In1), EPR2_sensor/1(In1)
  EGT/1 -> EGT_sensor/1(In1)  "EGT"
  CabinPressure/1 -> CabinPressure_sensor/1(In1)
  CabinPressure_sensor/1(Out1) -> Bus Creator7/2  "CabinPressure"
  LandingGearLeftLock/1 -> Data Type Conversion/1  "LandingGear"
  LandingGearLeftLock_sensor/1(Out1) -> Bus Creator7/5  "LGLeftLock"
  APUData/1 -> APUData_sensor/1(In1)
  APUData_sensor/1(Out1) -> Bus Creator7/4  "APUData"
  HydraulicPressure/1 -> HydraulicPressure_sensor/1(In1)
  HydraulicPressure_sensor/1(Out1) -> Bus Creator7/3  "HydraulicPressure"
  EPR1_sensor/1(Out1) -> Bus Creator6/6  "EPR1"
  EPR2_sensor/1(Out1) -> Bus Creator6/7  "EPR2"
  OilPressure/1 -> OilPressure_sensor/1(In1)  "oilpressure"
  OilPressure_sensor/1(Out1) -> Bus Creator6/4  "oilpressure"
  FuelPressure/1 -> FuelPressure_sensor/1(In1)  "fuelpressure"
  FuelPressure_sensor/1(Out1) -> Bus Creator6/3  "fuelpressure"
  RPM/1 -> RPM_sensor/1(In1)  "RPM"
  RPM_sensor/1(Out1) -> Bus Creator6/1  "RPM"
  Temperature_sensor/1(Out1) -> Bus Creator6/2  "temperature"
  SelectedHeading_sensor/1(Out1) -> Bus Creator5/4
  GroundSpeed_sensor/1(Out1) -> Bus Creator5/3
  Distance_sensor/1(Out1) -> Bus Creator5/2
  Bearing_sensor/1(Out1) -> Bus Creator5/1
  FlightAttitude_sensor/1(Out1) -> Bus Creator4/6
  RateOfTurn_sensor/1(Out1) -> Bus Creator4/5
  Altitude_sensor/1(Out1) -> Bus Creator4/4
  AirSpeed_sensor/1(Out1) -> Bus Creator4/3
  VerticalSpeed_sensor/1(Out1) -> Bus Creator4/2
  AirplaneDirection_sensor/1(Out1) -> Bus Creator4/1
  EGT_sensor/1(Out1) -> Bus Creator6/5  "EGT"
  FlapPosition_sensor/1(Out1) -> Bus Creator7/1  "FlapPosition"
  FuelQuantity/1 -> FuelQuantity_sensor/1(In1)  "FuelQuantity"
  FuelQuantity_sensor/1(Out1) -> Bus Creator6/8  "FuelQuantity"
  Data Type Conversion/1 -> LandingGearLeftLock_sensor/1(In1)
  LandingGearRightLock/1 -> Data Type Conversion1/1  "LandingGear"
  LandingGearRightLock_sensor/1(Out1) -> Bus Creator7/6  "LGRightLock"
  In1/1 -> RateOfTurn/1, AirSpeed/1, VerticalSpeed/1, AirplaneDirection/1, Altitude/1, FlightAttitude/1, Bearing/1, Distance/1, GroundSpeed/1, SelectedHeading/1, FuelQuantity/1, "FlapPosition "/1, APUData/1, LandingGearRightLock/1, LandingGearLeftLock/1, HydraulicPressure/1, CabinPressure/1, EPR/1, EGT/1, OilPressure/1, FuelPressure/1, Temperature/1, RPM/1
  Data Type Conversion1/1 -> LandingGearRightLock_sensor/1(In1)

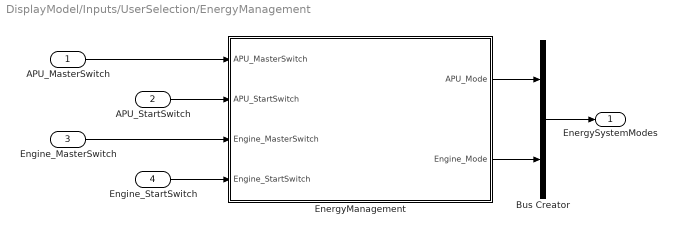
== system DisplayModel/Inputs/UserSelection/EnergyManagement ==
  APU_MasterSwitch : Inport
  APU_StartSwitch : Inport  Port=2
  Engine_MasterSwitch : Inport  Port=3
  Engine_StartSwitch : Inport  Port=4
  Bus Creator : BusCreator  Inputs=2
  EnergyManagement : Stateflow chart  TreatAsAtomicUnit=on
  EnergySystemModes : Outport
  wires:
  APU_MasterSwitch/1 -> EnergyManagement/1(APU_MasterSwitch)
  APU_StartSwitch/1 -> EnergyManagement/2(APU_StartSwitch)
  EnergyManagement/1(APU_Mode) -> Bus Creator/1
  EnergyManagement/2(Engine_Mode) -> Bus Creator/2
  Bus Creator/1 -> EnergySystemModes/1
  Engine_MasterSwitch/1 -> EnergyManagement/3(Engine_MasterSwitch)
  Engine_StartSwitch/1 -> EnergyManagement/4(Engine_StartSwitch)

== system DisplayModel/Inputs/UserSelection/NDAdditionalInput ==
  ARPT : Constant  Value=0  OutDataTypeStr=double
  Bus Creator : BusCreator  Inputs=5
  CSTR : Constant  Value=0  OutDataTypeStr=double
  NDB : Constant  Value=0  OutDataTypeStr=double
  VORD : Constant  Value=0  OutDataTypeStr=double
  WPT : Constant  Value=0  OutDataTypeStr=double
  Out1 : Outport
  wires:
  Bus Creator/1 -> Out1/1
  VORD/1 -> Bus Creator/3  "VORD"
  WPT/1 -> Bus Creator/2  "WPT"
  NDB/1 -> Bus Creator/4  "NDB"
  CSTR/1 -> Bus Creator/1  "CSTR"
  ARPT/1 -> Bus Creator/5  "ARPT"

== system DisplayModel/Control_and_Display_Logic/SignalConditioning/SignalSelection/DataValidityLandingGearLeftLock ==
  input signals : Inport  PortDimensions=3
  Range Threshold : Subsystem  RequirementInfo={} %GIDa_9464ebc1_75a4_4fc1_b22e_333f2b8b1e7f
  Screen Signals : Subsystem
  validated sensor : Outport
  wires:
  Range Threshold/1(Validity) -> Screen Signals/2(Validity)
  Screen Signals/1(validated sensor value) -> validated sensor/1
  input signals/1 -> Screen Signals/1(signals), Range Threshold/1(signals)

== system DisplayModel/Control_and_Display_Logic/SignalConditioning/SignalSelection/DataValidityLandingGearRightLock ==
  input signals : Inport  PortDimensions=3
  Range Threshold : Subsystem
  Screen Signals : Subsystem
  validated sensor : Outport
  wires:
  input signals/1 -> Range Threshold/1(signals), Screen Signals/1(signals)
  Screen Signals/1(validated sensor value) -> validated sensor/1
  Range Threshold/1(Validity) -> Screen Signals/2(Validity)

== system DisplayModel/Inputs/Sensors/SwitchedOff/APUData_sensor ==
  In1 : Inport
  Sensor_DataConversion : CockpitDisplayLib/Sensor_DataConversion  noise_factor=1
  Out1 : Outport
  wires:
  In1/1 -> Sensor_DataConversion/1  "APUData"
  Sensor_DataConversion/1 -> Out1/1

== system DisplayModel/Inputs/Sensors/SwitchedOff/AirSpeed_sensor ==
  In1 : Inport
  Out1 : Outport
  wires:
  In1/1 -> Out1/1

== system DisplayModel/Inputs/Sensors/SwitchedOff/AirplaneDirection_sensor ==
  In1 : Inport
  Out1 : Outport
  wires:
  In1/1 -> Out1/1

== system DisplayModel/Inputs/Sensors/SwitchedOff/Altitude_sensor ==
  In1 : Inport
  Out1 : Outport
  wires:
  In1/1 -> Out1/1

== system DisplayModel/Inputs/Sensors/SwitchedOff/Bearing_sensor ==
  In1 : Inport
  Out1 : Outport
  wires:
  In1/1 -> Out1/1

== system DisplayModel/Inputs/Sensors/SwitchedOff/CabinPressure_sensor ==
  In1 : Inport
  Sensor_DataConversion : CockpitDisplayLib/Sensor_DataConversion  noise_factor=0
  Out1 : Outport
  wires:
  In1/1 -> Sensor_DataConversion/1  "CabinPressure"
  Sensor_DataConversion/1 -> Out1/1

== system DisplayModel/Inputs/Sensors/SwitchedOff/Distance_sensor ==
  In1 : Inport
  Out1 : Outport
  wires:
  In1/1 -> Out1/1

== system DisplayModel/Inputs/Sensors/SwitchedOff/EGT_sensor ==
  In1 : Inport
  Sensor_DataConversion : CockpitDisplayLib/Sensor_DataConversion  noise_factor=0
  Out1 : Outport
  wires:
  In1/1 -> Sensor_DataConversion/1  "EGT"
  Sensor_DataConversion/1 -> Out1/1

== system DisplayModel/Inputs/Sensors/SwitchedOff/EPR1_sensor ==
  In1 : Inport
  Noise : Constant  Value=0
  Sensor_DataConversion : CockpitDisplayLib/Sensor_DataConversion  noise_factor=0
  Sum : Sum  Inputs=|++
  Out1 : Outport
  wires:
  Sum/1 -> Sensor_DataConversion/1  "EPR1"
  Noise/1 -> Sum/2
  In1/1 -> Sum/1
  Sensor_DataConversion/1 -> Out1/1

== system DisplayModel/Inputs/Sensors/SwitchedOff/EPR2_sensor ==
  In1 : Inport
  Noise : Constant  Value=0
  Sensor_DataConversion : CockpitDisplayLib/Sensor_DataConversion  noise_factor=0
  Sum : Sum  Inputs=|++
  Out1 : Outport
  wires:
  Sum/1 -> Sensor_DataConversion/1  "EPR2"
  Noise/1 -> Sum/2
  In1/1 -> Sum/1
  Sensor_DataConversion/1 -> Out1/1

== system DisplayModel/Inputs/Sensors/SwitchedOff/FlapPosition_sensor ==
  In1 : Inport
  Out1 : Outport
  wires:
  In1/1 -> Out1/1  "FlapPosition"

== system DisplayModel/Inputs/Sensors/SwitchedOff/FlightAttitude_sensor ==
  In1 : Inport
  Out1 : Outport
  wires:
  In1/1 -> Out1/1

== system DisplayModel/Inputs/Sensors/SwitchedOff/FuelPressure_sensor ==
  In1 : Inport
  Sensor_DataConversion : CockpitDisplayLib/Sensor_DataConversion  noise_factor=1
  Out1 : Outport
  wires:
  Sensor_DataConversion/1 -> Out1/1
  In1/1 -> Sensor_DataConversion/1

== system DisplayModel/Inputs/Sensors/SwitchedOff/FuelQuantity_sensor ==
  In1 : Inport
  Sensor_DataConversion : CockpitDisplayLib/Sensor_DataConversion  noise_factor=1
  Out1 : Outport
  wires:
  In1/1 -> Sensor_DataConversion/1  "FuelQuantity"
  Sensor_DataConversion/1 -> Out1/1

== system DisplayModel/Inputs/Sensors/SwitchedOff/GroundSpeed_sensor ==
  In1 : Inport
  Out1 : Outport
  wires:
  In1/1 -> Out1/1

== system DisplayModel/Inputs/Sensors/SwitchedOff/HydraulicPressure_sensor ==
  In1 : Inport
  Sensor_DataConversion : CockpitDisplayLib/Sensor_DataConversion  noise_factor=1
  Out1 : Outport
  wires:
  In1/1 -> Sensor_DataConversion/1  "HydraulicPressure"
  Sensor_DataConversion/1 -> Out1/1

== system DisplayModel/Inputs/Sensors/SwitchedOff/LandingGearLeftLock_sensor ==
  In1 : Inport
  ErrorValue : Constant  Value=0  OutDataTypeStr=boolean
  LGLeftLockFault_UserInput : Constant  Value=0
  Multiport Switch : MultiPortSwitch  DataPortOrder=Zero-based contiguous  Inputs=2
  Sensor_DataConversion : Subsystem  mask{noise_factor=1}
      mask prompts: noise_factor "noise factor"
      mask Callback noise_factor: noise_factor = 1;
  Out1 : Outport
  wires:
  Multiport Switch/1 -> Sensor_DataConversion/1(In1)  "LandingGear"
  In1/1 -> Multiport Switch/2
  LGLeftLockFault_UserInput/1 -> Multiport Switch/1
  ErrorValue/1 -> Multiport Switch/3
  Sensor_DataConversion/1(Out1) -> Out1/1

== system DisplayModel/Inputs/Sensors/SwitchedOff/LandingGearRightLock_sensor ==
  In1 : Inport
  ErrorValue : Constant  OutDataTypeStr=boolean
  LGLeftLockFault_UserInput : Constant  Value=0
  Multiport Switch : MultiPortSwitch  DataPortOrder=Zero-based contiguous  Inputs=2
  Sensor_DataConversion : Subsystem  mask{noise_factor=1}
      mask prompts: noise_factor "noise factor"
      mask Callback noise_factor: noise_factor = 1;
  Out1 : Outport
  wires:
  Sensor_DataConversion/1(Out1) -> Out1/1
  ErrorValue/1 -> Multiport Switch/3
  LGLeftLockFault_UserInput/1 -> Multiport Switch/1
  In1/1 -> Multiport Switch/2
  Multiport Switch/1 -> Sensor_DataConversion/1(In1)  "LandingGear"

== system DisplayModel/Inputs/Sensors/SwitchedOff/OilPressure_sensor ==
  In1 : Inport
  Sensor_DataConversion : CockpitDisplayLib/Sensor_DataConversion  noise_factor=0
  Out1 : Outport
  wires:
  Sensor_DataConversion/1 -> Out1/1  "oilpressure"
  In1/1 -> Sensor_DataConversion/1

== system DisplayModel/Inputs/Sensors/SwitchedOff/RPM_sensor ==
  In1 : Inport
  Sensor_DataConversion : CockpitDisplayLib/Sensor_DataConversion  noise_factor=0
  Out1 : Outport
  wires:
  In1/1 -> Sensor_DataConversion/1
  Sensor_DataConversion/1 -> Out1/1  "RPM"

== system DisplayModel/Inputs/Sensors/SwitchedOff/RateOfTurn_sensor ==
  In1 : Inport
  Out1 : Outport
  wires:
  In1/1 -> Out1/1

== system DisplayModel/Inputs/Sensors/SwitchedOff/SelectedHeading_sensor ==
  In1 : Inport
  Out1 : Outport
  wires:
  In1/1 -> Out1/1

== system DisplayModel/Inputs/Sensors/SwitchedOff/Temperature_sensor ==
  In1 : Inport
  Sensor_DataConversion : CockpitDisplayLib/Sensor_DataConversion  noise_factor=1
  Out1 : Outport
  wires:
  In1/1 -> Sensor_DataConversion/1
  Sensor_DataConversion/1 -> Out1/1

== system DisplayModel/Inputs/Sensors/SwitchedOff/VerticalSpeed_sensor ==
  In1 : Inport
  Out1 : Outport
  wires:
  In1/1 -> Out1/1

== system DisplayModel/Inputs/Sensors/SwitchedOn/APUData_sensor ==
  In1 : Inport
  APUFault_UserInput : Constant  Value=0
  ErrorValue : Constant  Value=0
  Multiport Switch : MultiPortSwitch  DataPortOrder=Zero-based contiguous  Inputs=2
  Sensor_DataConversion : CockpitDisplayLib/Sensor_DataConversion  noise_factor=1
  Out1 : Outport
  wires:
  Multiport Switch/1 -> Sensor_DataConversion/1  "APUData"
  APUFault_UserInput/1 -> Multiport Switch/1
  ErrorValue/1 -> Multiport Switch/3
  In1/1 -> Multiport Switch/2
  Sensor_DataConversion/1 -> Out1/1

== system DisplayModel/Inputs/Sensors/SwitchedOn/AirSpeed_sensor ==
  In1 : Inport
  Out1 : Outport
  wires:
  In1/1 -> Out1/1

== system DisplayModel/Inputs/Sensors/SwitchedOn/AirplaneDirection_sensor ==
  In1 : Inport
  Out1 : Outport
  wires:
  In1/1 -> Out1/1

== system DisplayModel/Inputs/Sensors/SwitchedOn/Altitude_sensor ==
  In1 : Inport
  Out1 : Outport
  wires:
  In1/1 -> Out1/1

== system DisplayModel/Inputs/Sensors/SwitchedOn/Bearing_sensor ==
  In1 : Inport
  Out1 : Outport
  wires:
  In1/1 -> Out1/1

== system DisplayModel/Inputs/Sensors/SwitchedOn/CabinPressure_sensor ==
  In1 : Inport
  CabinLowPrFault_UserInput : Constant  Value=0
  ErrorValue : Constant  Value=0
  Multiport Switch : MultiPortSwitch  DataPortOrder=Zero-based contiguous  Inputs=2
  Sensor_DataConversion : CockpitDisplayLib/Sensor_DataConversion  noise_factor=1
  Out1 : Outport
  wires:
  CabinLowPrFault_UserInput/1 -> Multiport Switch/1
  In1/1 -> Multiport Switch/2
  ErrorValue/1 -> Multiport Switch/3
  Multiport Switch/1 -> Sensor_DataConversion/1  "CabinPressure"
  Sensor_DataConversion/1 -> Out1/1

== system DisplayModel/Inputs/Sensors/SwitchedOn/Distance_sensor ==
  In1 : Inport
  Out1 : Outport
  wires:
  In1/1 -> Out1/1

== system DisplayModel/Inputs/Sensors/SwitchedOn/EGT_sensor ==
  In1 : Inport
  Sensor_DataConversion : CockpitDisplayLib/Sensor_DataConversion  noise_factor=0
  Out1 : Outport
  wires:
  In1/1 -> Sensor_DataConversion/1  "EGT"
  Sensor_DataConversion/1 -> Out1/1

== system DisplayModel/Inputs/Sensors/SwitchedOn/EPR1_sensor ==
  In1 : Inport
  Noise : Constant  Value=0
  Sensor_DataConversion : CockpitDisplayLib/Sensor_DataConversion  noise_factor=0
  Sum : Sum  Inputs=|++
  Out1 : Outport
  wires:
  Sum/1 -> Sensor_DataConversion/1  "EPR1"
  Noise/1 -> Sum/2
  In1/1 -> Sum/1
  Sensor_DataConversion/1 -> Out1/1  "EPR1"

== system DisplayModel/Inputs/Sensors/SwitchedOn/EPR2_sensor ==
  In1 : Inport
  Noise : Constant  Value=0
  Sensor_DataConversion : CockpitDisplayLib/Sensor_DataConversion  noise_factor=0
  Sum1 : Sum  Inputs=|++
  Out1 : Outport
  wires:
  Sum1/1 -> Sensor_DataConversion/1  "EPR2"
  Noise/1 -> Sum1/2
  In1/1 -> Sum1/1
  Sensor_DataConversion/1 -> Out1/1  "EPR2"

== system DisplayModel/Inputs/Sensors/SwitchedOn/FlapPosition_sensor ==
  In1 : Inport
  Out1 : Outport
  wires:
  In1/1 -> Out1/1  "FlapPosition"

== system DisplayModel/Inputs/Sensors/SwitchedOn/FlightAttitude_sensor ==
  In1 : Inport
  Out1 : Outport
  wires:
  In1/1 -> Out1/1

== system DisplayModel/Inputs/Sensors/SwitchedOn/FuelPressure_sensor ==
  In1 : Inport
  ErrorValue : Constant  Value=0
  FuelLowPrFault_UserInput : Constant  Value=0
  Multiport Switch : MultiPortSwitch  DataPortOrder=Zero-based contiguous  Inputs=2
  Sensor_DataConversion : CockpitDisplayLib/Sensor_DataConversion  noise_factor=1
  Out1 : Outport
  wires:
  FuelLowPrFault_UserInput/1 -> Multiport Switch/1
  Multiport Switch/1 -> Sensor_DataConversion/1  "fuelflow"
  In1/1 -> Multiport Switch/2
  ErrorValue/1 -> Multiport Switch/3
  Sensor_DataConversion/1 -> Out1/1

== system DisplayModel/Inputs/Sensors/SwitchedOn/FuelQuantity_sensor ==
  In1 : Inport
  Constant6 : Constant  Value=0
  FuelQnttyLowFault_UserInput : Constant  Value=0
  Multiport Switch : MultiPortSwitch  DataPortOrder=Zero-based contiguous  Inputs=2
  Sensor_DataConversion : CockpitDisplayLib/Sensor_DataConversion  noise_factor=0.001
  Out1 : Outport
  wires:
  In1/1 -> Multiport Switch/2
  FuelQnttyLowFault_UserInput/1 -> Multiport Switch/1
  Constant6/1 -> Multiport Switch/3
  Multiport Switch/1 -> Sensor_DataConversion/1  "FuelQuantity"
  Sensor_DataConversion/1 -> Out1/1

== system DisplayModel/Inputs/Sensors/SwitchedOn/GroundSpeed_sensor ==
  In1 : Inport
  Out1 : Outport
  wires:
  In1/1 -> Out1/1

== system DisplayModel/Inputs/Sensors/SwitchedOn/HydraulicPressure_sensor ==
  In1 : Inport
  ErrorValue : Constant  Value=0
  HydLowPrFault_UserInput : Constant  Value=0
  Multiport Switch : MultiPortSwitch  DataPortOrder=Zero-based contiguous  Inputs=2
  Sensor_DataConversion : CockpitDisplayLib/Sensor_DataConversion  noise_factor=1
  Out1 : Outport
  wires:
  Multiport Switch/1 -> Sensor_DataConversion/1  "HydraulicPressure"
  HydLowPrFault_UserInput/1 -> Multiport Switch/1
  ErrorValue/1 -> Multiport Switch/3
  In1/1 -> Multiport Switch/2
  Sensor_DataConversion/1 -> Out1/1

== system DisplayModel/Inputs/Sensors/SwitchedOn/LandingGearLeftLock_sensor ==
  In1 : Inport
  ErrorValue : Constant  Value=0  OutDataTypeStr=boolean
  LGLeftLockFault_UserInput : Constant  Value=0
  Multiport Switch : MultiPortSwitch  DataPortOrder=Zero-based contiguous  Inputs=2
  Sensor_DataConversion : Subsystem  mask{noise_factor=1}
      mask prompts: noise_factor "noise factor"
      mask Callback noise_factor: noise_factor = 1;
  Out1 : Outport
  wires:
  Multiport Switch/1 -> Sensor_DataConversion/1(In1)  "LandingGear"
  In1/1 -> Multiport Switch/2
  LGLeftLockFault_UserInput/1 -> Multiport Switch/1
  ErrorValue/1 -> Multiport Switch/3
  Sensor_DataConversion/1(Out1) -> Out1/1

== system DisplayModel/Inputs/Sensors/SwitchedOn/LandingGearRightLock_sensor ==
  In1 : Inport
  ErrorValue : Constant  OutDataTypeStr=boolean
  LGRightLockFault_UserInput : Constant  Value=0
  Multiport Switch : MultiPortSwitch  DataPortOrder=Zero-based contiguous  Inputs=2
  Sensor_DataConversion : Subsystem  mask{noise_factor=1}
      mask prompts: noise_factor "noise factor"
      mask Callback noise_factor: noise_factor = 1;
  Out1 : Outport
  wires:
  Sensor_DataConversion/1(Out1) -> Out1/1
  ErrorValue/1 -> Multiport Switch/3
  LGRightLockFault_UserInput/1 -> Multiport Switch/1
  In1/1 -> Multiport Switch/2
  Multiport Switch/1 -> Sensor_DataConversion/1(In1)  "LandingGear"

== system DisplayModel/Inputs/Sensors/SwitchedOn/OilPressure_sensor ==
  In1 : Inport
  EngineOilLowPrFault_UserInput : Constant  Value=0
  ErrorValue : Constant  Value=0
  Multiport Switch : MultiPortSwitch  DataPortOrder=Zero-based contiguous  Inputs=2
  Sensor_DataConversion : CockpitDisplayLib/Sensor_DataConversion  noise_factor=0.001
  Out1 : Outport
  wires:
  In1/1 -> Multiport Switch/2
  EngineOilLowPrFault_UserInput/1 -> Multiport Switch/1
  ErrorValue/1 -> Multiport Switch/3
  Multiport Switch/1 -> Sensor_DataConversion/1  "oilpressure"
  Sensor_DataConversion/1 -> Out1/1

== system DisplayModel/Inputs/Sensors/SwitchedOn/RPM_sensor ==
  In1 : Inport
  EngineSpeedFault_UserInput : Constant  Value=0
  ErrorValue : Constant  Value=0
  Multiport Switch : MultiPortSwitch  DataPortOrder=Zero-based contiguous  Inputs=2
  Sensor_DataConversion : CockpitDisplayLib/Sensor_DataConversion  noise_factor=0
  Out1 : Outport
  wires:
  EngineSpeedFault_UserInput/1 -> Multiport Switch/1
  ErrorValue/1 -> Multiport Switch/3
  In1/1 -> Multiport Switch/2
  Multiport Switch/1 -> Sensor_DataConversion/1
  Sensor_DataConversion/1 -> Out1/1  "RPM"

== system DisplayModel/Inputs/Sensors/SwitchedOn/RateOfTurn_sensor ==
  In1 : Inport
  Out1 : Outport
  wires:
  In1/1 -> Out1/1

== system DisplayModel/Inputs/Sensors/SwitchedOn/SelectedHeading_sensor ==
  In1 : Inport
  Out1 : Outport
  wires:
  In1/1 -> Out1/1

== system DisplayModel/Inputs/Sensors/SwitchedOn/Temperature_sensor ==
  In1 : Inport
  Sensor_DataConversion : CockpitDisplayLib/Sensor_DataConversion  noise_factor=1
  Out1 : Outport
  wires:
  In1/1 -> Sensor_DataConversion/1
  Sensor_DataConversion/1 -> Out1/1

== system DisplayModel/Inputs/Sensors/SwitchedOn/VerticalSpeed_sensor ==
  In1 : Inport
  Out1 : Outport
  wires:
  In1/1 -> Out1/1

== system DisplayModel/Control_and_Display_Logic/SignalConditioning/SignalSelection/DataValidityLandingGearLeftLock/Range Threshold ==
  note: This test checks whether the signals are within
      | the normal bounds of the sensor
  signals : Inport
  Logical Operator : Logic  AllPortsSameDT=off
  Relational Operator : RelationalOperator  Operator=<
  Relational Operator1 : RelationalOperator  Operator=>
  pos_max : Constant  Value=1.5
  pos_min : Constant  Value=-0.5
  Validity : Outport
  wires:
  signals/1 -> Relational Operator/1, Relational Operator1/1
  Relational Operator/1 -> Logical Operator/1
  Relational Operator1/1 -> Logical Operator/2
  pos_max/1 -> Relational Operator/2
  pos_min/1 -> Relational Operator1/2
  Logical Operator/1 -> Validity/1

== system DisplayModel/Control_and_Display_Logic/SignalConditioning/SignalSelection/DataValidityLandingGearLeftLock/Screen Signals ==
  signals : Inport
  Validity : Inport  Port=2
  Chart (MATLAB) : Stateflow chart  TreatAsAtomicUnit=on
  Data Type Conversion : DataTypeConversion  OutDataTypeStr=double
  validated sensor value : Outport
  wires:
  Data Type Conversion/1 -> Chart (MATLAB)/2(validity)
  signals/1 -> Chart (MATLAB)/1(signals)
  Validity/1 -> Data Type Conversion/1
  Chart (MATLAB)/1(valid_signal) -> validated sensor value/1
